simulink model "stepandfangbo"  (R2018a)
settings: Solver=VariableStepAuto  StartTime=0.0  StopTime=30  RelTol=1e-3
settings Model: Creator=Administrator  LastModifiedBy=Administrator

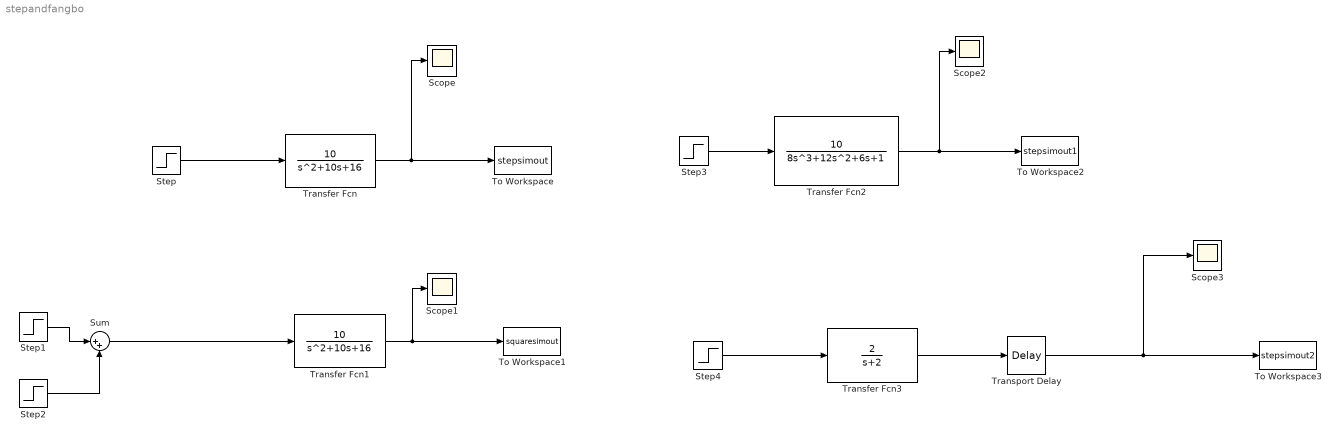
== system stepandfangbo ==
  Scope{,1..3} (4 alike) : Scope
  Step{,1,3..4} (4 alike) : Step  Time=0  After=2  SampleTime=0
  Step2 : Step  Time=4  After=-2  SampleTime=0
  Sum : Sum  Inputs=|++
  To Workspace : ToWorkspace  VariableName=stepsimout  SampleTime=0.2
      settings: Save2DSignal=2-D array (concatenate along first dimension)
  To Workspace1 : ToWorkspace  VariableName=squaresimout  SampleTime=0.2
      settings: Save2DSignal=2-D array (concatenate along first dimension)
  To Workspace2 : ToWorkspace  VariableName=stepsimout1  SampleTime=0.2
      settings: Save2DSignal=2-D array (concatenate along first dimension)
  To Workspace3 : ToWorkspace  VariableName=stepsimout2  SampleTime=0.2
      settings: Save2DSignal=2-D array (concatenate along first dimension)
  Transfer Fcn : TransferFcn  Numerator=[10]  Denominator=[1 10 16]
  Transfer Fcn1 : TransferFcn  Numerator=[10]  Denominator=[1 10 16]
  Transfer Fcn2 : TransferFcn  Numerator=[10]  Denominator=[8 12 6 1]
  Transfer Fcn3 : TransferFcn  Numerator=[2]  Denominator=[1 2]
  Transport Delay : TransportDelay  DelayTime=2
  wires:
  Step/1 -> Transfer Fcn/1
  Transfer Fcn/1 -> To Workspace/1, Scope/1
  Transfer Fcn1/1 -> To Workspace1/1, Scope1/1
  Step2/1 -> Sum/2
  Step1/1 -> Sum/1
  Sum/1 -> Transfer Fcn1/1
  Transfer Fcn2/1 -> To Workspace2/1, Scope2/1
  Step3/1 -> Transfer Fcn2/1
  Step4/1 -> Transfer Fcn3/1
  Transport Delay/1 -> Scope3/1, To Workspace3/1
  Transfer Fcn3/1 -> Transport Delay/1
